simulink model "QPSK2"  (R2017a)
settings: Solver=VariableStepAuto  StartTime=0.0  StopTime=10.0  RelTol=1e-3
libraries: commutil2 x2, dsparch4 x2, dspsigops x2, commchan3 x1, commrandsrc3 x1, commsink2 x1, dspindex x1
settings Model: Creator=81228  LastModifiedBy=81228

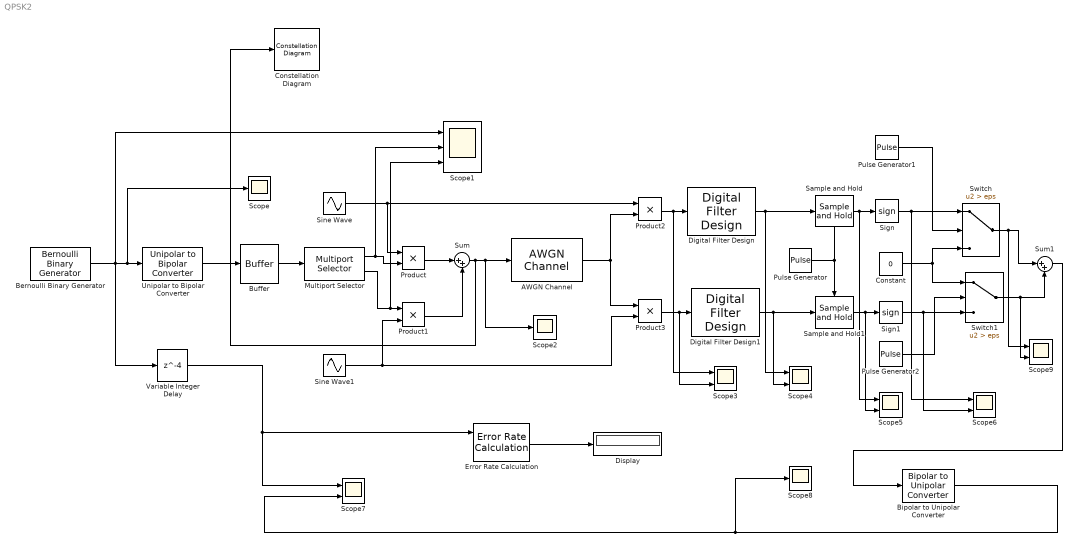
== system QPSK2 ==
  AWGN Channel : commchan3/AWGN Channel  InputProcessing=Inherited (this choice will be removed - see release notes)  seed=67  noiseMode=Variance from mask  EbNodB=10  EsNodB=10  SNRdB=10  bitsPerSym=1  Ps=1  Tsym=1  variance=0.01
  Bernoulli Binary Generator : commrandsrc3/Bernoulli Binary Generator  ProbabilityOfZero=0.5  SeedSource=Parameter  Seed=61  SampleTime=0.01  SamplesPerFrame=1  OutputDataType=double  SimulateUsing=Interpreted execution
  Bipolar to Unipolar Converter : commutil2/Bipolar to Unipolar Converter  M=4  polarity=Positive  dataType=Inherit via internal rule
      settings: SourceProductName=Communications System Toolbox  SourceProductBaseCode=CM
  Buffer : Buffer  N=2  OutputFrames=off
  Constant : Constant  Value=0
  Constellation Diagram : ConstellationDiagram
  Digital Filter Design : dsparch4/Digital Filter Design  mwdsp_browser_bugfix_var=off
  Digital Filter Design1 : dsparch4/Digital Filter Design  mwdsp_browser_bugfix_var=off
  Display : Display
  Error Rate Calculation : commsink2/Error Rate Calculation  N=0  st_delay=0  cp_mode=Entire frame  subframe=[]  PMode=Port  WsName=ErrorVec  RsMode2=off  stop=off  numErr=100  maxBits=1e6
  Multiport Selector : dspindex/Multiport Selector  rowsOrCols=Rows  idxCellArray={1,2}  idxErrMode=Clip Index
  Product{,1..3} (4 alike) : Product
  Pulse Generator : DiscretePulseGenerator  PulseWidth=2  PhaseDelay=2
  Pulse Generator1 : DiscretePulseGenerator  PulseWidth=2  PhaseDelay=2
  Pulse Generator2 : DiscretePulseGenerator  PulseWidth=2  PhaseDelay=2
  Sample and Hold : dspsigops/Sample and Hold  trig=Rising edge  initCond=0  latchinput=off
  Sample and Hold1 : dspsigops/Sample and Hold  trig=Rising edge  initCond=0  latchinput=off
  Scope : Scope
  Scope1 : Scope  NumInputPorts=3
  Scope2 : Scope
  Scope{3..7,9} (6 alike) : Scope  NumInputPorts=2
  Scope8 : Scope
  Sign : Signum
  Sign1 : Signum
  Sine Wave : Sin  Amplitude=2  Frequency=1000*pi  Phase=pi/2  SampleTime=1/10000
  Sine Wave1 : Sin  Amplitude=2  Frequency=1000*pi  Phase=pi/2  SampleTime=1/10000
  Sum : Sum  Inputs=|++
  Sum1 : Sum  Inputs=|++
  Switch : Switch  Criteria=u2 > Threshold  Threshold=eps
  Switch1 : Switch  Criteria=u2 > Threshold  Threshold=eps
  Unipolar to Bipolar Converter : commutil2/Unipolar to Bipolar Converter  M=2  polarity=Positive  dataType=Inherit via internal rule
      settings: SourceProductName=Communications System Toolbox
  Variable Integer Delay : Delay  DelayLength=4
  wires:
  Bernoulli Binary Generator/1 -> Variable Integer Delay/1, Scope1/1, Scope/1, Unipolar to Bipolar Converter/1
  Unipolar to Bipolar Converter/1 -> Buffer/1
  Sum/1 -> Constellation Diagram/1, Scope2/1, AWGN Channel/1
  Product/1 -> Sum/1
  Product1/1 -> Sum/2
  Sine Wave1/1 -> Product3/2, Product1/2
  Buffer/1 -> Multiport Selector/1
  Sine Wave/1 -> Product/1, Product2/1
  AWGN Channel/1 -> Product3/1, Product2/2
  Variable Integer Delay/1 -> Error Rate Calculation/1, Scope7/1
  Error Rate Calculation/1 -> Display/1
  Product2/1 -> Scope3/1, Digital Filter Design/1
  Product3/1 -> Scope3/2, Digital Filter Design1/1
  Digital Filter Design/1 -> Scope4/1, Sample and Hold/1
  Digital Filter Design1/1 -> Scope4/2, Sample and Hold1/1
  Sample and Hold/1 -> Scope5/1, Sign/1
  Sample and Hold1/1 -> Scope5/2, Sign1/1
  Sign/1 -> Scope6/1, Switch/1
  Pulse Generator1/1 -> Switch/2
  Constant/1 -> Switch1/1, Switch/3
  Sign1/1 -> Scope6/2, Switch1/3
  Pulse Generator2/1 -> Switch1/2
  Switch/1 -> Scope9/1, Sum1/1
  Switch1/1 -> Scope9/2, Sum1/2
  Pulse Generator/1 -> Sample and Hold1/Trigger, Sample and Hold/Trigger
  Sum1/1 -> Bipolar to Unipolar Converter/1
  Bipolar to Unipolar Converter/1 -> Scope8/1, Scope7/2
  Multiport Selector/2 -> Scope1/3, Product1/1
  Multiport Selector/1 -> Scope1/2, Product/2
